simulink model "OFDM_Tx_HW"  (R2020a)
settings: Solver=FixedStepDiscrete  StartTime=0.0  StopTime=inf  RelTol=1e-3
InitFcn:
  | % Set parameters
  | fs = 20e6;
  | fclk = 240e6;
  | ssr = 2;
  | fdc = fclk*ssr*8;
  | 
  | % Load libraries
  | addpath('./lib');
  | 
  | % Create filters
  | run ./filter_design_20mhz;
  | 
  | % Load all required variables
  | load('variables/read_addr_data');
  | load('variables/read_addr_cp');
  | load('variables/read_addr_pream');
  | load('variables/read_addr_rx');
  | load('variables/pilot');
  | load('variables/sc_index');
  | load('variables/LTSfreq');
  | load('variables/STSfreq');
  | load('variables/LTSread');
  | load('variables/STSread');
  | 
  | run ./scripts/rfgen;
values from neighbouring files (symbols this model uses):
  decimation_unique = dsp.SampleRateConverter('InputSampleRate', fdc/64,     'OutputSampleRate', fs,     'Bandwidth', fs*0.9,     'OutputRateTolerance', 0,     'StopbandAttenuation', 100)    [filter_design_20mhz.m]
  interpolation_single = dsp.SampleRateConverter('InputSampleRate', fs,     'OutputSampleRate', fclk,     'Bandwidth', fs*0.9,     'OutputRateTolerance', 0,     'StopbandAttenuation', 100)    [filter_design_20mhz.m]
  interpolation_ssr = dsp.SampleRateConverter('InputSampleRate', fclk,     'OutputSampleRate', fclk*ssr,     'Bandwidth', fs*0.9,     'OutputRateTolerance', 0,     'StopbandAttenuation', 100)    [filter_design_20mhz.m]
undefined symbols (not defined in the file or in its folder): designMultirateFIR, LTSfreq, LTSread, pilot, read_addr_cp, read_addr_data, read_addr_pream, read_addr_rx, sc_index, STSfreq, STSread
libraries: hdlsllib x87, simulink x55, xbsIndex_r4 x48, dspmlti4 x23, xrbsSSR_Library x8, dspsigops x6, dspswit3 x4, dsphdlmathfun x3, dspsigattribs x2, dsphdlxfrm x2, dsphdlsigops x1, lib_rfsignalgenerator x1
(part 3 of 6)

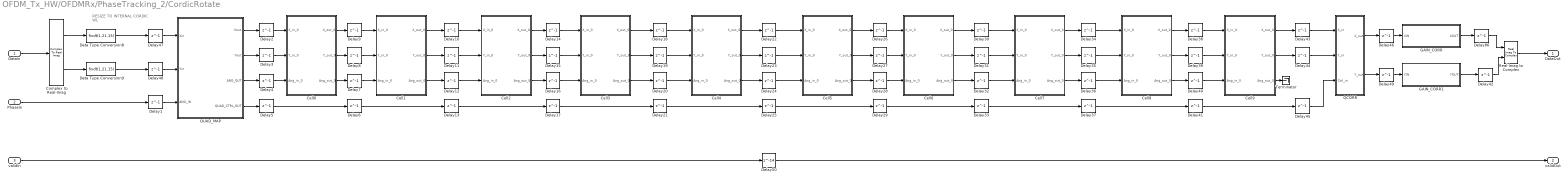
== system OFDM_Tx_HW/OFDMRx/PhaseTracking_2/CordicRotate ==
  note: RESIZE TO INTERNAL
      | CORDIC WL
  DataIn : Inport
  PhaseIn : Inport  Port=2
  validIn : Inport  Port=3
  Cell0 : Subsystem
  Cell1 : Subsystem
  Cell2 : Subsystem
  Cell3 : Subsystem
  Cell4 : Subsystem
  Cell5 : Subsystem
  Cell6 : Subsystem
  Cell7 : Subsystem
  Cell8 : Subsystem
  Cell9 : Subsystem
  Complex to Real-Imag : ComplexToRealImag
  Data Type Conversion8 : DataTypeConversion  OutDataTypeStr=fixdt(1,21,15)
  Data Type Conversion9 : DataTypeConversion  OutDataTypeStr=fixdt(1,21,15)
  Delay{1..49,86} (50 alike) : Delay  DelayLength=1
  Delay50 : Delay  DelayLength=14
  GAIN_CORR : Subsystem
  GAIN_CORR1 : Subsystem
  QCORR : Subsystem
  QUAD_MAP : Subsystem
  Real-Imag to Complex : RealImagToComplex
  Terminator : Terminator
  "DataOut  " : Outport  VectorParamsAs1DForOutWhenUnconnected=off
  validOut : Outport  Port=2  VectorParamsAs1DForOutWhenUnconnected=off
  wires:
  Delay50/1 -> validOut/1
  validIn/1 -> Delay50/1
  Real-Imag to Complex/1 -> "DataOut  "/1
  Delay42/1 -> Real-Imag to Complex/2
  Delay86/1 -> Real-Imag to Complex/1
  Complex to Real-Imag/1 -> Data Type Conversion8/1
  DataIn/1 -> Complex to Real-Imag/1
  Complex to Real-Imag/2 -> Data Type Conversion9/1
  GAIN_CORR/1(XOUT) -> Delay86/1
  Delay48/1 -> QUAD_MAP/2(Yin)
  Delay47/1 -> QUAD_MAP/1(Xin)
  QUAD_MAP/1(Xout) -> Delay2/1
  QUAD_MAP/2(Yout) -> Delay3/1
  QUAD_MAP/3(ANG_OUT) -> Delay4/1
  Delay2/1 -> Cell0/1(X_in_0)
  Delay3/1 -> Cell0/2(Y_in_0)
  QUAD_MAP/4(QUAD_CTRL_OUT) -> Delay5/1
  Cell0/1(X_out_0) -> Delay9/1
  Cell0/2(Y_out_0) -> Delay8/1
  Cell0/3(Ang_out_0) -> Delay7/1
  Delay5/1 -> Delay6/1
  Delay7/1 -> Cell1/3(Ang_in_0)
  Delay8/1 -> Cell1/2(Y_in_0)
  Delay9/1 -> Cell1/1(X_in_0)
  Cell1/1(X_out_0) -> Delay10/1
  Cell1/2(Y_out_0) -> Delay11/1
  Cell1/3(Ang_out_0) -> Delay12/1
  Delay6/1 -> Delay13/1
  Delay10/1 -> Cell2/1(X_in_0)
  Delay11/1 -> Cell2/2(Y_in_0)
  Delay12/1 -> Cell2/3(Ang_in_0)
  Delay16/1 -> Cell3/3(Ang_in_0)
  Delay15/1 -> Cell3/2(Y_in_0)
  Delay14/1 -> Cell3/1(X_in_0)
  Delay13/1 -> Delay17/1
  Cell2/3(Ang_out_0) -> Delay16/1
  Cell2/2(Y_out_0) -> Delay15/1
  Cell2/1(X_out_0) -> Delay14/1
  Cell3/1(X_out_0) -> Delay18/1
  Cell3/2(Y_out_0) -> Delay19/1
  Cell3/3(Ang_out_0) -> Delay20/1
  Delay17/1 -> Delay21/1
  Delay18/1 -> Cell4/1(X_in_0)
  Delay19/1 -> Cell4/2(Y_in_0)
  Delay20/1 -> Cell4/3(Ang_in_0)
  Delay24/1 -> Cell5/3(Ang_in_0)
  Delay23/1 -> Cell5/2(Y_in_0)
  Delay22/1 -> Cell5/1(X_in_0)
  Delay21/1 -> Delay25/1
  Cell4/3(Ang_out_0) -> Delay24/1
  Cell4/2(Y_out_0) -> Delay23/1
  Cell4/1(X_out_0) -> Delay22/1
  Cell5/1(X_out_0) -> Delay26/1
  Cell5/2(Y_out_0) -> Delay27/1
  Cell5/3(Ang_out_0) -> Delay28/1
  Delay25/1 -> Delay29/1
  Delay26/1 -> Cell6/1(X_in_0)
  Delay27/1 -> Cell6/2(Y_in_0)
  Delay28/1 -> Cell6/3(Ang_in_0)
  Delay32/1 -> Cell7/3(Ang_in_0)
  Delay31/1 -> Cell7/2(Y_in_0)
  Delay30/1 -> Cell7/1(X_in_0)
  Delay29/1 -> Delay33/1
  Cell6/3(Ang_out_0) -> Delay32/1
  Cell6/2(Y_out_0) -> Delay31/1
  Cell6/1(X_out_0) -> Delay30/1
  Cell7/1(X_out_0) -> Delay34/1
  Cell7/2(Y_out_0) -> Delay35/1
  Cell7/3(Ang_out_0) -> Delay36/1
  Delay33/1 -> Delay37/1
  Delay34/1 -> Cell8/1(X_in_0)
  Delay35/1 -> Cell8/2(Y_in_0)
  Delay36/1 -> Cell8/3(Ang_in_0)
  Delay40/1 -> Cell9/3(Ang_in_0)
  Delay39/1 -> Cell9/2(Y_in_0)
  Delay38/1 -> Cell9/1(X_in_0)
  Delay37/1 -> Delay41/1
  Cell8/3(Ang_out_0) -> Delay40/1
  Cell8/2(Y_out_0) -> Delay39/1
  Cell8/1(X_out_0) -> Delay38/1
  GAIN_CORR1/1(YOUT) -> Delay42/1
  Cell9/3(Ang_out_0) -> Terminator/1
  Delay41/1 -> Delay45/1
  Cell9/1(X_out_0) -> Delay43/1
  Cell9/2(Y_out_0) -> Delay44/1
  Delay43/1 -> QCORR/1(X_in)
  Delay44/1 -> QCORR/2(Y_in)
  Delay46/1 -> GAIN_CORR/1(XIN)
  Delay49/1 -> GAIN_CORR1/1(YIN)
  QCORR/2(Y_out) -> Delay49/1
  Delay1/1 -> QUAD_MAP/3(ANG_IN)
  Delay4/1 -> Cell0/3(Ang_in_0)
  Delay45/1 -> QCORR/3(Ctrl_in)
  Data Type Conversion8/1 -> Delay47/1
  Data Type Conversion9/1 -> Delay48/1
  PhaseIn/1 -> Delay1/1
  QCORR/1(X_out) -> Delay46/1

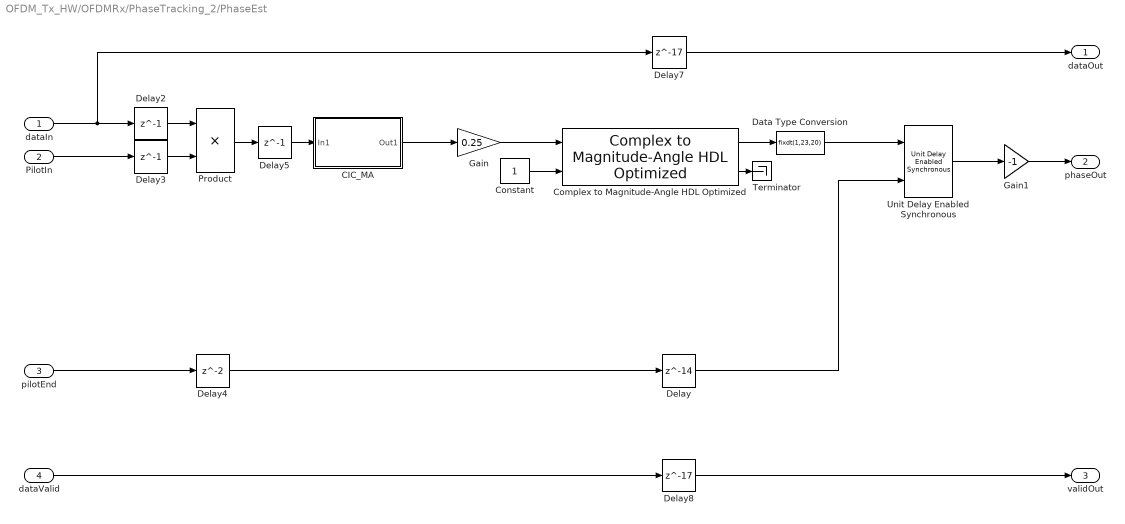
== system OFDM_Tx_HW/OFDMRx/PhaseTracking_2/PhaseEst ==
  dataIn : Inport
  PilotIn : Inport  Port=2
  pilotEnd : Inport  Port=3
  dataValid : Inport  Port=4
  CIC_MA : Subsystem
  Complex to Magnitude-Angle HDL Optimized : dsphdlmathfun/Complex to Magnitude-Angle HDL Optimized  NumIterationsSource=Property  NumIterations=10  OutputFormat=Angle  AngleFormat=Radians  ScaleOutput=off  SimulateUsing=Code generation
      settings: SourceProductBaseCode=DS
  Constant : Constant  OutDataTypeStr=boolean  SampleTime=1/fs
  Data Type Conversion : DataTypeConversion  OutDataTypeStr=fixdt(1,23,20)
  Delay : Delay  DelayLength=14
  Delay2 : Delay  DelayLength=1
  Delay3 : Delay  DelayLength=1
  Delay4 : Delay
  Delay5 : Delay  DelayLength=1
  Delay7 : Delay  DelayLength=17
  Delay8 : Delay  DelayLength=17
  Gain : Gain  Gain=0.25  OutDataTypeStr=fixdt(1,18,15)
  Gain1 : Gain  Gain=-1  OutDataTypeStr=fixdt(1,23,20)
  Product : Product  OutDataTypeStr=fixdt(1,18,15)
  Terminator : Terminator
  Unit Delay Enabled Synchronous : hdlsllib/Discrete/Unit Delay Enabled Synchronous  InitialCondition=0.0  SampleTime=-1
      settings: SourceProductBaseCode=SL
  dataOut : Outport  VectorParamsAs1DForOutWhenUnconnected=off
  phaseOut : Outport  Port=2  VectorParamsAs1DForOutWhenUnconnected=off
  validOut : Outport  Port=3  VectorParamsAs1DForOutWhenUnconnected=off
  wires:
  Data Type Conversion/1 -> Unit Delay Enabled Synchronous/1
  Gain1/1 -> phaseOut/1
  Delay4/1 -> Delay/1
  Complex to Magnitude-Angle HDL Optimized/2 -> Terminator/1
  Complex to Magnitude-Angle HDL Optimized/1 -> Data Type Conversion/1
  Gain/1 -> Complex to Magnitude-Angle HDL Optimized/1
  Constant/1 -> Complex to Magnitude-Angle HDL Optimized/2
  Delay8/1 -> validOut/1
  Unit Delay Enabled Synchronous/1 -> Gain1/1
  Delay7/1 -> dataOut/1
  dataValid/1 -> Delay8/1
  pilotEnd/1 -> Delay4/1
  Delay5/1 -> CIC_MA/1(In1)
  Delay3/1 -> Product/2
  Delay2/1 -> Product/1
  Product/1 -> Delay5/1
  dataIn/1 -> Delay2/1, Delay7/1
  PilotIn/1 -> Delay3/1
  Delay/1 -> Unit Delay Enabled Synchronous/2
  CIC_MA/1(Out1) -> Gain/1

== system OFDM_Tx_HW/OFDMRx/PhaseTracking_2/PilotCtrlGen ==
  dataIn : Inport
  ValidIn : Inport  Port=2
  CtrlSigGen : Subsystem
  Delay1 : Delay  DelayLength=1
  Delay10 : Delay  DelayLength=1
  SampleCounter : Subsystem
  SymbolCounter : Subsystem
  pilotGen : Subsystem
  dataOut : Outport  VectorParamsAs1DForOutWhenUnconnected=off
  pilotOut : Outport  Port=2  VectorParamsAs1DForOutWhenUnconnected=off
  PilotEnd : Outport  Port=3  VectorParamsAs1DForOutWhenUnconnected=off
  dataValid : Outport  Port=4  VectorParamsAs1DForOutWhenUnconnected=off
  wires:
  Delay1/1 -> pilotGen/3(valid), CtrlSigGen/1(valid)
  SampleCounter/1(Sample_Cnt) -> pilotGen/2(sampleCount), CtrlSigGen/2(sampleCount)
  CtrlSigGen/2(pilotEnd) -> PilotEnd/1
  CtrlSigGen/1(dataValid) -> dataValid/1
  SymbolCounter/1(Symbl_cnt) -> pilotGen/1(symbCount)
  ValidIn/1 -> SymbolCounter/1(ValidIn), SampleCounter/1(Valid_In), Delay1/1
  pilotGen/1(pilOut) -> pilotOut/1
  Delay10/1 -> dataOut/1
  dataIn/1 -> Delay10/1

== system OFDM_Tx_HW/OFDMRx/Synchronisation/CoarseFreqCorr ==
  note: Reccord the phase of the averaged autocorrelation at the coarse
      | timing point.
  note: Correct frequency offset
  note: Generate complex sinusoid with a frequency equal
      | to the estimated frequency offset.
  dataIn : Inport
  frameDet : Inport  Port=2
  phaseIn : Inport  Port=3
  Constant : Constant  VectorParams1D=off  OutDataTypeStr=boolean  SampleTime=1/fs
  Delay{,2,5,7} (4 alike) : Delay  DelayLength=1
  Delay1 : Delay  DelayLength=9
  Delay3 : Delay  DelayLength=6
  Gain : Gain  Gain=2048  OutDataTypeStr=uint16
  Math Function : Math  Operator=conj  SignedPower=on  RndMeth=Zero  SaturateOnIntegerOverflow=on
  NCO HDL Optimized : dsphdlsigops/NCO HDL Optimized  PhaseIncrementSource=Input port  PhaseIncrement=100  PhaseOffsetSource=Property  PhaseOffset=0  DitherSource=Property  NumDitherBits=4  SamplesPerFrame=1  LUTCompress=on  ResetAction=off  Waveform=Complex exponential  PhasePort=off  SimulateUsing=Code generation  AccumulatorWL=16  PhaseQuantization=on  NumQuantizerAccumulatorBits=12  OutputDataType=Binary point scaling  OutputWL=16  OutputFL=14
      settings: SourceProductBaseCode=DS
  Product : Product  OutDataTypeStr=fixdt(1,16,14)
  RsingEdge : Subsystem
  Terminator : Terminator
  Unit Delay Enabled Synchronous : hdlsllib/Discrete/Unit Delay Enabled Synchronous  InitialCondition=0.0  SampleTime=-1
      settings: SourceProductBaseCode=SL
  dataOut : Outport  VectorParamsAs1DForOutWhenUnconnected=off
  frameDetOut : Outport  Port=2  VectorParamsAs1DForOutWhenUnconnected=off
  wires:
  Delay7/1 -> dataOut/1
  Delay1/1 -> frameDetOut/1
  Math Function/1 -> Delay5/1
  Delay3/1 -> Delay/1
  Product/1 -> Delay7/1
  Delay5/1 -> Product/2
  Delay/1 -> Product/1
  dataIn/1 -> Delay2/1
  phaseIn/1 -> Unit Delay Enabled Synchronous/1
  RsingEdge/1(Out1) -> Unit Delay Enabled Synchronous/2
  frameDet/1 -> Delay1/1, RsingEdge/1(In1)
  Delay2/1 -> Delay3/1
  Unit Delay Enabled Synchronous/1 -> Gain/1
  Gain/1 -> NCO HDL Optimized/1
  NCO HDL Optimized/1 -> Math Function/1
  NCO HDL Optimized/2 -> Terminator/1
  Constant/1 -> NCO HDL Optimized/2

== system OFDM_Tx_HW/OFDMRx/Synchronisation/ControlSigGen ==
  validIn : Inport
  OR : Logic  Operator=OR  IconShape=distinctive  AllPortsSameDT=off  OutDataTypeStr=boolean
  PreambleValidGen : Subsystem
  dataValidGen : Subsystem
  FFTValid : Outport  VectorParamsAs1DForOutWhenUnconnected=off
  dataValid : Outport  Port=2  VectorParamsAs1DForOutWhenUnconnected=off
  preambleValid : Outport  Port=3  VectorParamsAs1DForOutWhenUnconnected=off
  wires:
  OR/1 -> FFTValid/1
  dataValidGen/1(y) -> dataValid/1, OR/2
  PreambleValidGen/1(y) -> dataValidGen/1(enb), OR/1, preambleValid/1
  validIn/1 -> PreambleValidGen/1(ValidIn), dataValidGen/2(enb1)

== system OFDM_Tx_HW/OFDMRx/Synchronisation/Delay ==
  note: Delay coarse timing point from middle of L-STF
      | to beginning of 1st repetition of L-LTF
  data : Inport
  strobe : Inport  Port=2
  Delay3 : Delay  DelayLength=108  InputProcessing=Columns as channels (frame based)
  dataOut : Outport
  strobeOut : Outport  Port=2
  wires:
  data/1 -> dataOut/1
  Delay3/1 -> strobeOut/1
  strobe/1 -> Delay3/1

== system OFDM_Tx_HW/OFDMRx/Synchronisation/FrameDetect ==
  note: The frame is detected when the timing metric exceeds the threshold for 30 successive samples. This
      | corresponds to the coarse timing point, which should occur in the middle of the L-STF.
  leftIn : Inport
  rightIn : Inport  Port=2
  phaseIn : Inport  Port=3
  Compare To Constant : simulink/Logic and Bit Operations/Compare To Constant  relop===  const=29  OutDataTypeStr=boolean
  Delay{,2..4} (4 alike) : Delay  DelayLength=1
  HDL Counter : hdlsllib/Sources/HDL Counter  CountType=Count limited  CountInit=0  CountStep=1  CountMax=29  CountFromType=Initial value  CountFrom=0  CountResetPort=on  CountLoadPort=off  CountEnbPort=on  CountDirPort=off  CountDataType=Unsigned  CountWordLen=5  CountFracLen=0  CountSampTime=1
  Logical Operator : Logic  Operator=OR  IconShape=distinctive  AllPortsSameDT=off  OutDataTypeStr=boolean
  Logical Operator1 : Logic  Operator=NOT  IconShape=distinctive  AllPortsSameDT=off  OutDataTypeStr=boolean
  Relational Operator : RelationalOperator  Operator=>  OutDataTypeStr=boolean  RndMeth=Simplest
  RsingEdge : Subsystem
  frameDet : Outport  VectorParamsAs1DForOutWhenUnconnected=off
  phaseOut : Outport  Port=2  VectorParamsAs1DForOutWhenUnconnected=off
  wires:
  Delay3/1 -> Relational Operator/2
  Relational Operator/1 -> HDL Counter/2, Logical Operator1/1
  Logical Operator1/1 -> Logical Operator/2
  rightIn/1 -> Delay3/1
  HDL Counter/1 -> Compare To Constant/1
  Compare To Constant/1 -> RsingEdge/1(In1), Logical Operator/1
  Logical Operator/1 -> HDL Counter/1
  phaseIn/1 -> Delay4/1
  leftIn/1 -> Delay2/1
  Delay/1 -> phaseOut/1
  RsingEdge/1(Out1) -> frameDet/1
  Delay2/1 -> Relational Operator/1
  Delay4/1 -> Delay/1

== system OFDM_Tx_HW/OFDMRx/Synchronisation/SchmidlCoxMetric  ==
  note: The Schmidl & Cox timing metric is used for frame detection. The timing metric, M(d), is compared to a threshold
      | to determine if a frame is present. In order to avoid division, we re-arrange the timing metric as |P(d)|^2 > (R(d))^2 x thresh.
      | The phase of the averaged autocorrelation is also determined for Carrier Frequency Offset (CFO) estimation purposes.
  note: |P(d)|^2
  note: (R(d))^2 x thresh
  dataIn : Inport
  threshold : Inport  Port=2
  Abs2 : Subsystem
  AutoCorr : Subsystem
  CIC_ma : Subsystem
  CIC_ma1 : Subsystem
  Data Type Conversion : DataTypeConversion  OutDataTypeStr=fixdt(0,32,31)  ConvertRealWorld=Stored Integer (SI)
  Delay : Delay  DelayLength=14
  Delay2 : Delay
  MagPhase : Subsystem
  Sq : Subsystem
  Sq1 : Subsystem
  ThreshMult : Subsystem
  left : Outport  VectorParamsAs1DForOutWhenUnconnected=off
  right : Outport  Port=2  VectorParamsAs1DForOutWhenUnconnected=off
  phase : Outport  Port=3  VectorParamsAs1DForOutWhenUnconnected=off
  wires:
  threshold/1 -> Data Type Conversion/1
  Data Type Conversion/1 -> ThreshMult/2(threshold)
  Sq/1(Out1) -> left/1
  ThreshMult/1(Out1) -> right/1
  Sq1/1(Out1) -> ThreshMult/1(In1)
  Delay/1 -> Sq1/1(In1)
  CIC_ma1/1(Out1) -> Delay/1
  dataIn/1 -> AutoCorr/1(AcorrIn), Abs2/1(Abs2In)
  Abs2/1(Abs2Out) -> CIC_ma1/1(In1)
  MagPhase/2(Mag) -> Sq/1(In1)
  AutoCorr/1(AcorrOut) -> CIC_ma/1(In1)
  CIC_ma/1(Out1) -> MagPhase/1(dataIn)
  Delay2/1 -> phase/1
  MagPhase/1(Phase) -> Delay2/1

== system OFDM_Tx_HW/OFDMTx/CPAdd/DataExtend ==
  dataIn : Inport
  dataValid : Inport  Port=2
  Delay1 : Delay  DelayLength=80  InitialCondition=0  UseCircularBuffer=on
  Delay2 : Delay  DelayLength=80
  Delay3 : Delay  DelayLength=1  InitialCondition=0  UseCircularBuffer=on
  Delay4 : Delay  DelayLength=80
  Dual Port RAM2 : hdlsllib/HDL RAMs/Dual Port RAM  ram_size=8
      settings: SourceProductBaseCode=SL
  HDL Counter : hdlsllib/Sources/HDL Counter  CountType=Count limited  CountInit=0  CountStep=1  CountMax=159  CountFromType=Initial value  CountFrom=0  CountResetPort=off  CountLoadPort=off  CountEnbPort=on  CountDirPort=off  CountDataType=Unsigned  CountWordLen=8  CountFracLen=0  CountSampTime=1
  HDL Counter1 : hdlsllib/Sources/HDL Counter  CountType=Count limited  CountInit=0  CountStep=1  CountMax=159  CountFromType=Initial value  CountFrom=0  CountResetPort=off  CountLoadPort=off  CountEnbPort=on  CountDirPort=off  CountDataType=Unsigned  CountWordLen=8  CountFracLen=0  CountSampTime=1
  READ_ADDRESS : Lookup_n-D  NumberOfTableDimensions=1  LookupTableObject=''  BreakpointsForDimension1=[0:159]  BreakpointsForDimension1FirstPoint=10  BreakpointsForDimension2FirstPoint=10  BreakpointsForDimension1Spacing=12  BreakpointsForDimension2Spacing=12  IndexSearchMethod=Evenly spaced points  Table=read_addr_cp  TableDataTypeStr=fixdt(0,8,0)  InterpMethod=Flat  DiagnosticForOutOfRangeInput=Error  InternalRulePriority=Speed  OutDataTypeStr=fixdt(0,8,0)  RndMeth=Simplest  InputSameDT=on
  READ_CTRL2 : Subsystem
  Terminator3 : Terminator
  dataOut : Outport  VectorParamsAs1DForOutWhenUnconnected=off
  dataValidOut : Outport  Port=2  VectorParamsAs1DForOutWhenUnconnected=off
  wires:
  Delay4/1 -> dataOut/1
  Delay2/1 -> dataValidOut/1
  Dual Port RAM2/1 -> Terminator3/1
  READ_ADDRESS/1 -> READ_CTRL2/1(In1)
  HDL Counter/1 -> READ_ADDRESS/1
  dataIn/1 -> Dual Port RAM2/1
  HDL Counter1/1 -> Dual Port RAM2/2
  Delay1/1 -> HDL Counter/1, Delay3/1, READ_CTRL2/2(In2)
  Dual Port RAM2/2 -> Delay4/1
  dataValid/1 -> HDL Counter1/1, Dual Port RAM2/3, Delay1/1
  Delay3/1 -> Delay2/1
  READ_CTRL2/1(Out1) -> Dual Port RAM2/4

== system OFDM_Tx_HW/OFDMTx/CPAdd/LTFExtend ==
  data : Inport
  preambVal : Inport  Port=2
  Delay : Delay  DelayLength=160  InitialCondition=0  UseCircularBuffer=on
  Delay12 : Delay  DelayLength=1  InitialCondition=0  UseCircularBuffer=on
  Dual Port RAM : hdlsllib/HDL RAMs/Dual Port RAM  ram_size=8
      settings: SourceProductBaseCode=SL
  HDL Counter2 : hdlsllib/Sources/HDL Counter  CountType=Count limited  CountInit=0  CountStep=1  CountMax=159  CountFromType=Initial value  CountFrom=0  CountResetPort=off  CountLoadPort=off  CountEnbPort=on  CountDirPort=off  CountDataType=Unsigned  CountWordLen=8  CountFracLen=0  CountSampTime=1
  HDL Counter3 : hdlsllib/Sources/HDL Counter  CountType=Count limited  CountInit=0  CountStep=1  CountMax=159  CountFromType=Initial value  CountFrom=0  CountResetPort=off  CountLoadPort=off  CountEnbPort=on  CountDirPort=off  CountDataType=Unsigned  CountWordLen=8  CountFracLen=0  CountSampTime=1
  LTFValidGen : Subsystem
  READ_CTRL : Subsystem
  Terminator1 : Terminator
  readaddr : Lookup_n-D  NumberOfTableDimensions=1  LookupTableObject=''  BreakpointsForDimension1=0:159  BreakpointsForDimension1FirstPoint=10  BreakpointsForDimension2FirstPoint=10  BreakpointsForDimension1Spacing=12  BreakpointsForDimension2Spacing=12  IndexSearchMethod=Evenly spaced points  Table=LTSread  TableDataTypeStr=fixdt(0,8,0)  InterpMethod=Flat  DiagnosticForOutOfRangeInput=Error  InternalRulePriority=Speed  OutDataTypeStr=fixdt(0,8,0)  RndMeth=Simplest  InputSameDT=on
  LTFExtendOut : Outport  VectorParamsAs1DForOutWhenUnconnected=off
  LTFValidOut : Outport  Port=2  VectorParamsAs1DForOutWhenUnconnected=off
  wires:
  readaddr/1 -> READ_CTRL/1(In1)
  READ_CTRL/1(Out1) -> Dual Port RAM/4
  HDL Counter3/1 -> Dual Port RAM/2
  Delay/1 -> READ_CTRL/2(In2), Delay12/1, HDL Counter2/1
  Dual Port RAM/1 -> Terminator1/1
  Delay12/1 -> LTFValidOut/1
  HDL Counter2/1 -> readaddr/1
  data/1 -> Dual Port RAM/1
  Dual Port RAM/2 -> LTFExtendOut/1
  preambVal/1 -> LTFValidGen/1(In1)
  LTFValidGen/1(Out1) -> Dual Port RAM/3, Delay/1, HDL Counter3/1

== system OFDM_Tx_HW/OFDMTx/CPAdd/STFExtend ==
  data : Inport
  preambVal : Inport  Port=2
  Delay : Delay  DelayLength=160  InitialCondition=0  UseCircularBuffer=on
  Delay12 : Delay  DelayLength=1  InitialCondition=0  UseCircularBuffer=on
  Dual Port RAM : hdlsllib/HDL RAMs/Dual Port RAM  ram_size=8
      settings: SourceProductBaseCode=SL
  HDL Counter2 : hdlsllib/Sources/HDL Counter  CountType=Count limited  CountInit=0  CountStep=1  CountMax=159  CountFromType=Initial value  CountFrom=0  CountResetPort=off  CountLoadPort=off  CountEnbPort=on  CountDirPort=off  CountDataType=Unsigned  CountWordLen=8  CountFracLen=0  CountSampTime=1
  HDL Counter3 : hdlsllib/Sources/HDL Counter  CountType=Count limited  CountInit=0  CountStep=1  CountMax=159  CountFromType=Initial value  CountFrom=0  CountResetPort=off  CountLoadPort=off  CountEnbPort=on  CountDirPort=off  CountDataType=Unsigned  CountWordLen=8  CountFracLen=0  CountSampTime=1
  READ_CTRL : Subsystem
  STFValidGen : Subsystem
  Terminator1 : Terminator
  readaddr : Lookup_n-D  NumberOfTableDimensions=1  LookupTableObject=''  BreakpointsForDimension1=0:159  BreakpointsForDimension1FirstPoint=10  BreakpointsForDimension2FirstPoint=10  BreakpointsForDimension1Spacing=12  BreakpointsForDimension2Spacing=12  IndexSearchMethod=Evenly spaced points  Table=STSread  TableDataTypeStr=fixdt(0,8,0)  InterpMethod=Flat  DiagnosticForOutOfRangeInput=Error  InternalRulePriority=Speed  OutDataTypeStr=fixdt(0,8,0)  RndMeth=Simplest  InputSameDT=on
  STFExtendOut : Outport  VectorParamsAs1DForOutWhenUnconnected=off
  STFValidOut : Outport  Port=2  VectorParamsAs1DForOutWhenUnconnected=off
  wires:
  Dual Port RAM/2 -> STFExtendOut/1
  data/1 -> Dual Port RAM/1
  HDL Counter2/1 -> readaddr/1
  Delay12/1 -> STFValidOut/1
  Dual Port RAM/1 -> Terminator1/1
  Delay/1 -> HDL Counter2/1, Delay12/1, READ_CTRL/2(In2)
  HDL Counter3/1 -> Dual Port RAM/2
  READ_CTRL/1(Out1) -> Dual Port RAM/4
  preambVal/1 -> STFValidGen/1(In1)
  readaddr/1 -> READ_CTRL/1(In1)
  STFValidGen/1(Out1) -> HDL Counter3/1, Dual Port RAM/3, Delay/1

== system OFDM_Tx_HW/OFDMTx/ControlSignalGenerator/PreamValidGen ==
  enable : Inport
  Compare To Constant : simulink/Logic and Bit Operations/Compare To Constant  relop===  const=320  OutDataTypeStr=boolean
  HDL Counter : hdlsllib/Sources/HDL Counter  CountType=Count limited  CountInit=0  CountStep=1  CountMax=320  CountFromType=Initial value  CountFrom=0  CountResetPort=on  CountLoadPort=off  CountEnbPort=on  CountDirPort=off  CountDataType=Unsigned  CountWordLen=9  CountFracLen=0  CountSampTime=1
  NOT : Logic  Operator=NOT  IconShape=distinctive  AllPortsSameDT=off  OutDataTypeStr=boolean
  RisingEdge : Subsystem
  Unit Delay Enabled Resettable Synchronous : hdlsllib/Discrete/Unit Delay Enabled Resettable Synchronous  InitialCondition=0.0  SampleTime=-1
      settings: SourceProductBaseCode=SL
  y : Outport  VectorParamsAs1DForOutWhenUnconnected=off
  wires:
  HDL Counter/1 -> Compare To Constant/1
  RisingEdge/1(Out1) -> Unit Delay Enabled Resettable Synchronous/2
  Compare To Constant/1 -> Unit Delay Enabled Resettable Synchronous/3
  enable/1 -> RisingEdge/1(In1), Unit Delay Enabled Resettable Synchronous/1, NOT/1, HDL Counter/2
  Unit Delay Enabled Resettable Synchronous/1 -> y/1
  NOT/1 -> HDL Counter/1

== system OFDM_Tx_HW/OFDMTx/ControlSignalGenerator/dataReadyGen ==
  enb : Inport
  Compare To Constant : simulink/Logic and Bit Operations/Compare To Constant  relop=>  const=31  OutDataTypeStr=boolean
  HDL Counter : hdlsllib/Sources/HDL Counter  CountType=Count limited  CountInit=0  CountStep=1  CountMax=79  CountFromType=Initial value  CountFrom=0  CountResetPort=on  CountLoadPort=off  CountEnbPort=on  CountDirPort=off  CountDataType=Unsigned  CountWordLen=7  CountFracLen=0  CountSampTime=1
  NOT : Logic  Operator=NOT  IconShape=distinctive  AllPortsSameDT=off  OutDataTypeStr=boolean
  y : Outport
  wires:
  HDL Counter/1 -> Compare To Constant/1
  enb/1 -> NOT/1, HDL Counter/2
  NOT/1 -> HDL Counter/1
  Compare To Constant/1 -> y/1

== system OFDM_Tx_HW/OFDMTx/ControlSignalGenerator/dataValidGen ==
  y : Inport
  enable : Inport  Port=2
  AND : Logic  IconShape=distinctive  AllPortsSameDT=off  OutDataTypeStr=boolean
  Delay : Delay  DelayLength=1
  NOT : Logic  Operator=NOT  IconShape=distinctive  AllPortsSameDT=off  OutDataTypeStr=boolean
  valOut : Outport
  wires:
  NOT/1 -> AND/1
  Delay/1 -> AND/2
  AND/1 -> valOut/1
  y/1 -> NOT/1
  enable/1 -> Delay/1

== system OFDM_Tx_HW/OFDMTx/ControlSignalGenerator/pilotValidGen ==
  enb : Inport
  AND : Logic  IconShape=distinctive  AllPortsSameDT=off  OutDataTypeStr=boolean
  Compare To Constant : simulink/Logic and Bit Operations/Compare To Constant  relop=<  const=32  OutDataTypeStr=boolean
  Compare To Constant1 : simulink/Logic and Bit Operations/Compare To Constant  relop=>  const=27  OutDataTypeStr=boolean
  HDL Counter : hdlsllib/Sources/HDL Counter  CountType=Count limited  CountInit=0  CountStep=1  CountMax=79  CountFromType=Initial value  CountFrom=0  CountResetPort=on  CountLoadPort=off  CountEnbPort=on  CountDirPort=off  CountDataType=Unsigned  CountWordLen=7  CountFracLen=0  CountSampTime=1
  NOT : Logic  Operator=NOT  IconShape=distinctive  AllPortsSameDT=off  OutDataTypeStr=boolean
  y : Outport
  wires:
  NOT/1 -> HDL Counter/1
  enb/1 -> HDL Counter/2, NOT/1
  HDL Counter/1 -> Compare To Constant1/1, Compare To Constant/1
  Compare To Constant/1 -> AND/1
  Compare To Constant1/1 -> AND/2
  AND/1 -> y/1

== system OFDM_Tx_HW/OFDMTx/DataGenerator/LTSfreq ==
  preambVal : Inport
  AND : Logic  IconShape=distinctive  AllPortsSameDT=off  OutDataTypeStr=boolean
  AND1 : Logic  IconShape=distinctive  AllPortsSameDT=off  OutDataTypeStr=boolean
  Compare To Constant : simulink/Logic and Bit Operations/Compare To Constant  relop=>=  const=256  OutDataTypeStr=boolean
  Compare To Constant1 : simulink/Logic and Bit Operations/Compare To Constant  relop=<=  const=319  OutDataTypeStr=boolean
  HDL Counter1 : hdlsllib/Sources/HDL Counter  CountType=Count limited  CountInit=0  CountStep=1  CountMax=319  CountFromType=Initial value  CountFrom=0  CountResetPort=on  CountLoadPort=off  CountEnbPort=on  CountDirPort=off  CountDataType=Unsigned  CountWordLen=9  CountFracLen=0  CountSampTime=1
  HDL Counter4 : hdlsllib/Sources/HDL Counter  CountType=Count limited  CountInit=0  CountStep=1  CountMax=63  CountFromType=Initial value  CountFrom=0  CountResetPort=off  CountLoadPort=off  CountEnbPort=on  CountDirPort=off  CountDataType=Unsigned  CountWordLen=6  CountFracLen=0  CountSampTime=1
  LTSFreq : Lookup_n-D  NumberOfTableDimensions=1  LookupTableObject=''  BreakpointsForDimension1=0:63  BreakpointsForDimension1FirstPoint=10  BreakpointsForDimension2FirstPoint=10  BreakpointsForDimension1Spacing=12  BreakpointsForDimension2Spacing=12  IndexSearchMethod=Evenly spaced points  Table=LTSfreq  TableDataTypeStr=fixdt(1,16,14)  InterpMethod=Flat  DiagnosticForOutOfRangeInput=Error  InternalRulePriority=Speed  OutDataTypeStr=fixdt(1,16,14)  RndMeth=Simplest  InputSameDT=on
  NOT : Logic  Operator=NOT  IconShape=distinctive  AllPortsSameDT=off  OutDataTypeStr=boolean
  ltsFreq : Outport  VectorParamsAs1DForOutWhenUnconnected=off
  ltsVal : Outport  Port=2  VectorParamsAs1DForOutWhenUnconnected=off
  wires:
  HDL Counter4/1 -> LTSFreq/1
  Compare To Constant/1 -> AND/1
  HDL Counter1/1 -> Compare To Constant1/1, Compare To Constant/1
  Compare To Constant1/1 -> AND/2
  NOT/1 -> HDL Counter1/1
  AND/1 -> AND1/1
  preambVal/1 -> NOT/1, AND1/2, HDL Counter1/2
  AND1/1 -> ltsVal/1, HDL Counter4/1
  LTSFreq/1 -> ltsFreq/1

== system OFDM_Tx_HW/OFDMTx/DataGenerator/PilotGen ==
  dataValidIn : Inport
  pilotValidIn : Inport  Port=2
  Compare To Constant : simulink/Logic and Bit Operations/Compare To Constant  relop=>  const=0  OutDataTypeStr=boolean
  Compare To Constant1 : simulink/Logic and Bit Operations/Compare To Constant  relop===  const=79  OutDataTypeStr=boolean
  Constant : Constant  Value=0  OutDataTypeStr=fixdt(1,2,0)  SampleTime=1/fs
  Data Type Conversion1 : DataTypeConversion  OutDataTypeStr=fixdt(1,16,14)
  HDL Counter : hdlsllib/Sources/HDL Counter  CountType=Count limited  CountInit=0  CountStep=1  CountMax=3  CountFromType=Initial value  CountFrom=0  CountResetPort=off  CountLoadPort=off  CountEnbPort=on  CountDirPort=off  CountDataType=Unsigned  CountWordLen=2  CountFracLen=0  CountSampTime=1
  HDL Counter1 : hdlsllib/Sources/HDL Counter  CountType=Count limited  CountInit=0  CountStep=1  CountMax=79  CountFromType=Initial value  CountFrom=0  CountResetPort=on  CountLoadPort=off  CountEnbPort=on  CountDirPort=off  CountDataType=Unsigned  CountWordLen=8  CountFracLen=0  CountSampTime=1
  HDL Counter2 : hdlsllib/Sources/HDL Counter  CountType=Count limited  CountInit=0  CountStep=1  CountMax=126  CountFromType=Initial value  CountFrom=0  CountResetPort=on  CountLoadPort=off  CountEnbPort=on  CountDirPort=off  CountDataType=Unsigned  CountWordLen=7  CountFracLen=0  CountSampTime=1
  NOT : Logic  Operator=NOT  IconShape=distinctive  AllPortsSameDT=off  OutDataTypeStr=boolean
  PilotValue_LUT : Lookup_n-D  NumberOfTableDimensions=1  LookupTableObject=''  BreakpointsForDimension1=[0:3]  BreakpointsForDimension1FirstPoint=10  BreakpointsForDimension2FirstPoint=10  BreakpointsForDimension1Spacing=12  BreakpointsForDimension2Spacing=12  IndexSearchMethod=Evenly spaced points  Table=[1 1 1 -1]  TableDataTypeStr=fixdt(1,2,0)  InterpMethod=Flat  DiagnosticForOutOfRangeInput=Error  InternalRulePriority=Speed  OutDataTypeStr=fixdt(1,2,0)  RndMeth=Simplest  InputSameDT=on
  Polarity_LUT : Lookup_n-D  NumberOfTableDimensions=1  LookupTableObject=''  BreakpointsForDimension1=[0:126]  BreakpointsForDimension1FirstPoint=10  BreakpointsForDimension2FirstPoint=10  BreakpointsForDimension1Spacing=12  BreakpointsForDimension2Spacing=12  IndexSearchMethod=Evenly spaced points  Table=pilot  TableDataTypeStr=fixdt(1,2,0)  InterpMethod=Flat  DiagnosticForOutOfRangeInput=Error  InternalRulePriority=Speed  OutDataTypeStr=fixdt(1,2,0)  RndMeth=Simplest  InputSameDT=on
  Switch : Switch  Criteria=u2 ~= 0
  Switch1 : Switch  Criteria=u2 ~= 0
  ToComplex1 : Subsystem
  Unary Minus : UnaryMinus
  pilotOut : Outport  VectorParamsAs1DForOutWhenUnconnected=off
  wires:
  HDL Counter/1 -> PilotValue_LUT/1
  Data Type Conversion1/1 -> ToComplex1/1(In1)
  dataValidIn/1 -> HDL Counter1/2, NOT/1
  HDL Counter1/1 -> Compare To Constant1/1
  NOT/1 -> HDL Counter2/1, HDL Counter1/1
  Compare To Constant1/1 -> HDL Counter2/2
  HDL Counter2/1 -> Polarity_LUT/1
  ToComplex1/1(PilotOut) -> pilotOut/1
  pilotValidIn/1 -> HDL Counter/1, Switch1/2
  Polarity_LUT/1 -> Compare To Constant/1
  Compare To Constant/1 -> Switch/2
  Unary Minus/1 -> Switch/3
  Switch/1 -> Data Type Conversion1/1
  PilotValue_LUT/1 -> Switch1/1
  Switch1/1 -> Unary Minus/1, Switch/1
  Constant/1 -> Switch1/3

== system OFDM_Tx_HW/OFDMTx/DataGenerator/STSFreq ==
  preamVal : Inport
  AND : Logic  IconShape=distinctive  AllPortsSameDT=off  OutDataTypeStr=boolean
  AND1 : Logic  IconShape=distinctive  AllPortsSameDT=off  OutDataTypeStr=boolean
  Compare To Constant : simulink/Logic and Bit Operations/Compare To Constant  relop=>=  const=96  OutDataTypeStr=boolean
  Compare To Constant1 : simulink/Logic and Bit Operations/Compare To Constant  relop=<=  const=159  OutDataTypeStr=boolean
  HDL Counter : hdlsllib/Sources/HDL Counter  CountType=Count limited  CountInit=0  CountStep=1  CountMax=63  CountFromType=Initial value  CountFrom=0  CountResetPort=off  CountLoadPort=off  CountEnbPort=on  CountDirPort=off  CountDataType=Unsigned  CountWordLen=6  CountFracLen=0  CountSampTime=1
  HDL Counter1 : hdlsllib/Sources/HDL Counter  CountType=Count limited  CountInit=0  CountStep=1  CountMax=319  CountFromType=Initial value  CountFrom=0  CountResetPort=on  CountLoadPort=off  CountEnbPort=on  CountDirPort=off  CountDataType=Unsigned  CountWordLen=9  CountFracLen=0  CountSampTime=1
  NOT : Logic  Operator=NOT  IconShape=distinctive  AllPortsSameDT=off  OutDataTypeStr=boolean
  STSFreq : Lookup_n-D  NumberOfTableDimensions=1  LookupTableObject=''  BreakpointsForDimension1=[0:63]  BreakpointsForDimension1FirstPoint=10  BreakpointsForDimension2FirstPoint=10  BreakpointsForDimension1Spacing=12  BreakpointsForDimension2Spacing=12  IndexSearchMethod=Evenly spaced points  Table=STSfreq  TableDataTypeStr=fixdt(1,16,14)  InterpMethod=Flat  DiagnosticForOutOfRangeInput=Error  InternalRulePriority=Speed  OutDataTypeStr=fixdt(1,16,14)  RndMeth=Simplest  InputSameDT=on
  stsFreq : Outport  VectorParamsAs1DForOutWhenUnconnected=off
  stsVal : Outport  Port=2  VectorParamsAs1DForOutWhenUnconnected=off
  wires:
  HDL Counter/1 -> STSFreq/1
  AND/1 -> AND1/1
  HDL Counter1/1 -> Compare To Constant1/1, Compare To Constant/1
  NOT/1 -> HDL Counter1/1
  Compare To Constant/1 -> AND/1
  Compare To Constant1/1 -> AND/2
  preamVal/1 -> NOT/1, AND1/2, HDL Counter1/2
  AND1/1 -> stsVal/1, HDL Counter/1
  STSFreq/1 -> stsFreq/1

== system OFDM_Tx_HW/OFDMTx/IFFT/IFFTValid ==
  preambleValid : Inport
  dataValid : Inport  Port=2
  Switch : Switch  Criteria=u2 ~= 0
  dataIFFTValid : Subsystem
  preambIFFTValid : Subsystem
  ifftValid : Outport  VectorParamsAs1DForOutWhenUnconnected=off
  wires:
  preambleValid/1 -> Switch/2, preambIFFTValid/1(preambValid)
  preambIFFTValid/1(preambIFFTValidOut) -> Switch/1
  dataValid/1 -> dataIFFTValid/1(dataValidIn)
  dataIFFTValid/1(dataIFFTValidOut) -> Switch/3
  Switch/1 -> ifftValid/1

== system OFDM_Tx_HW/OFDMTx/SCMapper/DataMapper ==
  dataIn : Inport
  dataValid : Inport  Port=2
  Delay1 : Delay  DelayLength=80  InitialCondition=0  UseCircularBuffer=on
  Delay2 : Delay  DelayLength=80
  Delay3 : Delay  DelayLength=1  InitialCondition=0  UseCircularBuffer=on
  Delay4 : Delay  DelayLength=80
  Dual Port RAM2 : hdlsllib/HDL RAMs/Dual Port RAM  ram_size=8
      settings: SourceProductBaseCode=SL
  HDL Counter : hdlsllib/Sources/HDL Counter  CountType=Count limited  CountInit=0  CountStep=1  CountMax=159  CountFromType=Initial value  CountFrom=0  CountResetPort=off  CountLoadPort=off  CountEnbPort=on  CountDirPort=off  CountDataType=Unsigned  CountWordLen=8  CountFracLen=0  CountSampTime=1
  HDL Counter1 : hdlsllib/Sources/HDL Counter  CountType=Count limited  CountInit=0  CountStep=1  CountMax=159  CountFromType=Initial value  CountFrom=0  CountResetPort=off  CountLoadPort=off  CountEnbPort=on  CountDirPort=off  CountDataType=Unsigned  CountWordLen=8  CountFracLen=0  CountSampTime=1
  READ_CTRL2 : Subsystem
  Terminator3 : Terminator
  readaddress : Lookup_n-D  NumberOfTableDimensions=1  LookupTableObject=''  BreakpointsForDimension1=[0:159]  BreakpointsForDimension1FirstPoint=10  BreakpointsForDimension2FirstPoint=10  BreakpointsForDimension1Spacing=12  BreakpointsForDimension2Spacing=12  IndexSearchMethod=Evenly spaced points  Table=read_addr_data  TableDataTypeStr=fixdt(0,8,0)  InterpMethod=Flat  DiagnosticForOutOfRangeInput=Error  InternalRulePriority=Speed  OutDataTypeStr=fixdt(0,8,0)  RndMeth=Simplest  InputSameDT=on
  dataOut : Outport  VectorParamsAs1DForOutWhenUnconnected=off
  dataValidOut : Outport  Port=2  VectorParamsAs1DForOutWhenUnconnected=off
  wires:
  READ_CTRL2/1(Out1) -> Dual Port RAM2/4
  Delay3/1 -> Delay2/1
  dataValid/1 -> HDL Counter1/1, Delay1/1, Dual Port RAM2/3
  Dual Port RAM2/2 -> Delay4/1
  Delay1/1 -> READ_CTRL2/2(In2), Delay3/1, HDL Counter/1
  HDL Counter1/1 -> Dual Port RAM2/2
  dataIn/1 -> Dual Port RAM2/1
  HDL Counter/1 -> readaddress/1
  readaddress/1 -> READ_CTRL2/1(In1)
  Dual Port RAM2/1 -> Terminator3/1
  Delay2/1 -> dataValidOut/1
  Delay4/1 -> dataOut/1

== system OFDM_Tx_HW/OFDMTx/SCMapper/PremableMapper ==
  data : Inport
  preambVal : Inport  Port=2
  Delay : Delay  DelayLength=160  InitialCondition=0  UseCircularBuffer=on
  Delay12 : Delay  DelayLength=1  InitialCondition=0  UseCircularBuffer=on
  Dual Port RAM : hdlsllib/HDL RAMs/Dual Port RAM  ram_size=9
      settings: SourceProductBaseCode=SL
  HDL Counter2 : hdlsllib/Sources/HDL Counter  CountType=Count limited  CountInit=0  CountStep=1  CountMax=319  CountFromType=Initial value  CountFrom=0  CountResetPort=off  CountLoadPort=off  CountEnbPort=on  CountDirPort=off  CountDataType=Unsigned  CountWordLen=9  CountFracLen=0  CountSampTime=1
  HDL Counter3 : hdlsllib/Sources/HDL Counter  CountType=Count limited  CountInit=0  CountStep=1  CountMax=319  CountFromType=Initial value  CountFrom=0  CountResetPort=off  CountLoadPort=off  CountEnbPort=on  CountDirPort=off  CountDataType=Unsigned  CountWordLen=9  CountFracLen=0  CountSampTime=1
  READ_CTRL : Subsystem
  Terminator1 : Terminator
  readaddr : Lookup_n-D  NumberOfTableDimensions=1  LookupTableObject=''  BreakpointsForDimension1=0:319  BreakpointsForDimension1FirstPoint=10  BreakpointsForDimension2FirstPoint=10  BreakpointsForDimension1Spacing=12  BreakpointsForDimension2Spacing=12  IndexSearchMethod=Evenly spaced points  Table=read_addr_pream  TableDataTypeStr=fixdt(0,9,0)  InterpMethod=Flat  DiagnosticForOutOfRangeInput=Error  InternalRulePriority=Speed  OutDataTypeStr=fixdt(0,9,0)  RndMeth=Simplest  InputSameDT=on
  preambleShiftOut : Outport  VectorParamsAs1DForOutWhenUnconnected=off
  preambValOut : Outport  Port=2  VectorParamsAs1DForOutWhenUnconnected=off
  wires:
  readaddr/1 -> READ_CTRL/1(In1)
  preambVal/1 -> Delay/1, Dual Port RAM/3, HDL Counter3/1
  READ_CTRL/1(Out1) -> Dual Port RAM/4
  HDL Counter3/1 -> Dual Port RAM/2
  Delay/1 -> READ_CTRL/2(In2), Delay12/1, HDL Counter2/1
  Dual Port RAM/1 -> Terminator1/1
  Delay12/1 -> preambValOut/1
  HDL Counter2/1 -> readaddr/1
  data/1 -> Dual Port RAM/1
  Dual Port RAM/2 -> preambleShiftOut/1

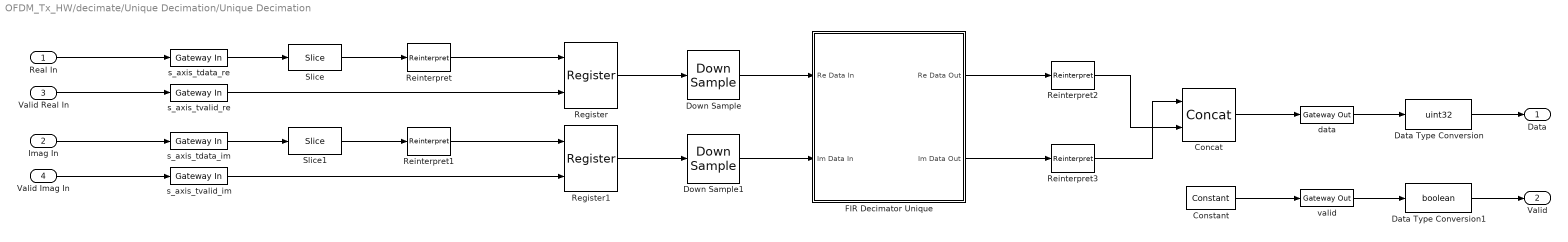
== system OFDM_Tx_HW/decimate/Unique Decimation/Unique Decimation ==
  Real In : Inport
  Imag In : Inport  Port=2
  Valid Real In : Inport  Port=3
  Valid Imag In : Inport  Port=4
  Concat : xbsIndex_r4/Concat  num_inputs=2  dbl_ovrd=off  block_type=concat
  Constant : xbsIndex_r4/Constant  const=1.0  gui_display_data_type=Boolean  arith_type=Boolean  n_bits=16  bin_pt=14  preci_type=Single  exp_width=8  frac_width=24  explicit_period=on  period=1/fs  equ=P=C  opselect=C  inp2=PCIN>>17  opr=+  inp1=P  carry=CIN  dbl_ovrd=off  block_type=constant
  Data Type Conversion : DataTypeConversion  OutDataTypeStr=uint32  ConvertRealWorld=Stored Integer (SI)
  Data Type Conversion1 : DataTypeConversion  OutDataTypeStr=boolean  ConvertRealWorld=Stored Integer (SI)
  Down Sample : xbsIndex_r4/Down Sample  sample_ratio=4  sample_phase="Last Value of Frame  (most efficient)"  en=off  rst=off  latency=1  dbl_ovrd=off  block_type=dsamp
  Down Sample1 : xbsIndex_r4/Down Sample  sample_ratio=4  sample_phase="Last Value of Frame  (most efficient)"  en=off  rst=off  latency=1  dbl_ovrd=off  block_type=dsamp
  FIR Decimator Unique : Subsystem
  Register : xbsIndex_r4/Register  init=0  rst=off  en=on  dbl_ovrd=off  block_type=register
  Register1 : xbsIndex_r4/Register  init=0  rst=off  en=on  dbl_ovrd=off  block_type=register
  Reinterpret : xbsIndex_r4/Reinterpret  force_arith_type=on  arith_type="Signed  (2's comp)"  force_bin_pt=on  bin_pt=14  block_type=reinterpret
  Reinterpret1 : xbsIndex_r4/Reinterpret  force_arith_type=on  arith_type="Signed  (2's comp)"  force_bin_pt=on  bin_pt=14  block_type=reinterpret
  Reinterpret2 : xbsIndex_r4/Reinterpret  force_arith_type=on  arith_type=Unsigned  force_bin_pt=on  bin_pt=0  block_type=reinterpret
  Reinterpret3 : xbsIndex_r4/Reinterpret  force_arith_type=on  arith_type=Unsigned  force_bin_pt=on  bin_pt=0  block_type=reinterpret
  Slice : xbsIndex_r4/Slice  nbits=1  boolean_output=off  mode=Two Bit Locations  bit1=15  base1=LSB of Input  bit0=0  base0=LSB of Input  dbl_ovrd=off  block_type=slice
  Slice1 : xbsIndex_r4/Slice  nbits=1  boolean_output=off  mode=Two Bit Locations  bit1=15  base1=LSB of Input  bit0=0  base0=LSB of Input  dbl_ovrd=off  block_type=slice
  data : xbsIndex_r4/Gateway Out  inherit_from_input=on  hdl_port=on  rows=1  columns=1  UseAsDAC=off  DACChannel='1'  interface=None  automatic_assignment=on  address_offset=hex2dec('00')  intf_name=''  intf_description=''  timing_constraint=None  locs_specified=off  LOCs={}  io_standard={}  block_type=gatewayout
  s_axis_tdata_im : xbsIndex_r4/Gateway In  gui_display_data_type=Fixed-point  arith_type=Unsigned  n_bits=128  bin_pt=0  preci_type=Single  exp_width=8  frac_width=24  rows=1  columns=1  quantization="Round  (unbiased: +/- Inf)"  overflow=Saturate  period=1/fclk  UseAsADC=off  ADCChannel='1'  interface=None  automatic_assignment=on  address_offset=hex2dec('00')  intf_name=''  intf_description=''  default_value=0  timing_constraint=None  locs_specified=off  LOCs={}  io_standard={}  inherit_from_input=off  hdl_port=on  dbl_ovrd=off  block_type=gatewayin
  s_axis_tdata_re : xbsIndex_r4/Gateway In  gui_display_data_type=Fixed-point  arith_type=Unsigned  n_bits=128  bin_pt=0  preci_type=Single  exp_width=8  frac_width=24  rows=1  columns=1  quantization="Round  (unbiased: +/- Inf)"  overflow=Saturate  period=1/fclk  UseAsADC=off  ADCChannel='1'  interface=None  automatic_assignment=on  address_offset=hex2dec('00')  intf_name=''  intf_description=''  default_value=0  timing_constraint=None  locs_specified=off  LOCs={}  io_standard={}  inherit_from_input=off  hdl_port=on  dbl_ovrd=off  block_type=gatewayin
  s_axis_tvalid_im : xbsIndex_r4/Gateway In  gui_display_data_type=Boolean  arith_type=Boolean  n_bits=16  bin_pt=14  preci_type=Single  exp_width=8  frac_width=24  rows=1  columns=1  quantization="Round  (unbiased: +/- Inf)"  overflow=Saturate  period=1/fclk  UseAsADC=off  ADCChannel='1'  interface=None  automatic_assignment=on  address_offset=hex2dec('00')  intf_name=''  intf_description=''  default_value=0  timing_constraint=None  locs_specified=off  LOCs={}  io_standard={}  inherit_from_input=off  hdl_port=on  dbl_ovrd=off  block_type=gatewayin
  s_axis_tvalid_re : xbsIndex_r4/Gateway In  gui_display_data_type=Boolean  arith_type=Boolean  n_bits=16  bin_pt=14  preci_type=Single  exp_width=8  frac_width=24  rows=1  columns=1  quantization="Round  (unbiased: +/- Inf)"  overflow=Saturate  period=1/fclk  UseAsADC=off  ADCChannel='1'  interface=None  automatic_assignment=on  address_offset=hex2dec('00')  intf_name=''  intf_description=''  default_value=0  timing_constraint=None  locs_specified=off  LOCs={}  io_standard={}  inherit_from_input=off  hdl_port=on  dbl_ovrd=off  block_type=gatewayin
  valid : xbsIndex_r4/Gateway Out  inherit_from_input=on  hdl_port=on  rows=1  columns=1  UseAsDAC=off  DACChannel='1'  interface=None  automatic_assignment=on  address_offset=hex2dec('00')  intf_name=''  intf_description=''  timing_constraint=None  locs_specified=off  LOCs={}  io_standard={}  block_type=gatewayout
  Data : Outport
  Valid : Outport  Port=2
  wires:
  Data Type Conversion1/1 -> Valid/1
  Data Type Conversion/1 -> Data/1
  Concat/1 -> data/1
  Reinterpret2/1 -> Concat/2
  Reinterpret3/1 -> Concat/1
  FIR Decimator Unique/2(Im Data Out) -> Reinterpret3/1
  FIR Decimator Unique/1(Re Data Out) -> Reinterpret2/1
  Constant/1 -> valid/1
  Real In/1 -> s_axis_tdata_re/1
  data/1 -> Data Type Conversion/1
  Reinterpret1/1 -> Register1/1
  s_axis_tdata_re/1 -> Slice/1
  Down Sample1/1 -> FIR Decimator Unique/2(Im Data In)
  Valid Real In/1 -> s_axis_tvalid_re/1
  Down Sample/1 -> FIR Decimator Unique/1(Re Data In)
  Imag In/1 -> s_axis_tdata_im/1
  Slice1/1 -> Reinterpret1/1
  Register1/1 -> Down Sample1/1
  s_axis_tvalid_im/1 -> Register1/2
  Reinterpret/1 -> Register/1
  valid/1 -> Data Type Conversion1/1
  Slice/1 -> Reinterpret/1
  s_axis_tvalid_re/1 -> Register/2
  s_axis_tdata_im/1 -> Slice1/1
  Valid Imag In/1 -> s_axis_tvalid_im/1
  Register/1 -> Down Sample/1

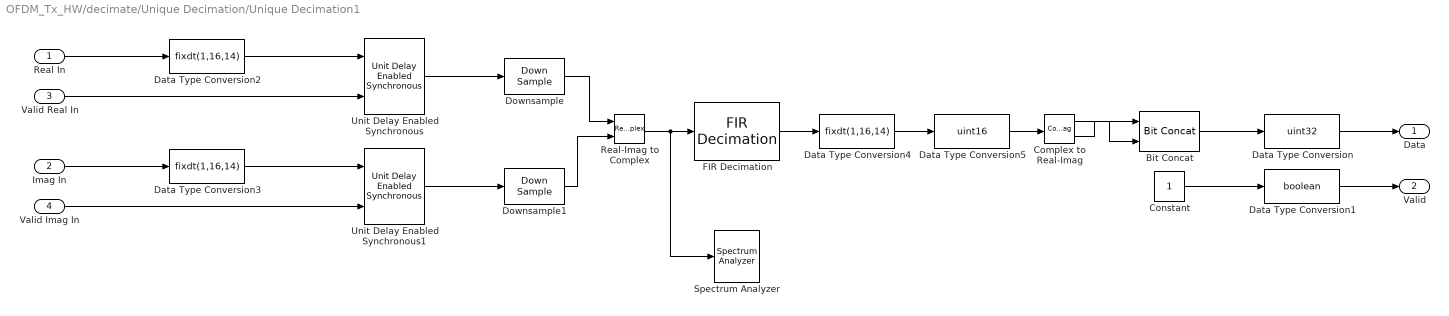
== system OFDM_Tx_HW/decimate/Unique Decimation/Unique Decimation1 ==
  Real In : Inport
  Imag In : Inport  Port=2
  Valid Real In : Inport  Port=3
  Valid Imag In : Inport  Port=4
  Bit Concat : hdlsllib/Logic and Bit Operations/Bit Concat  numInputs=2
  Complex to Real-Imag : ComplexToRealImag
  Constant : Constant  OutDataTypeStr=boolean  SampleTime=1/1e6
  Data Type Conversion : DataTypeConversion  OutDataTypeStr=uint32  ConvertRealWorld=Stored Integer (SI)
  Data Type Conversion1 : DataTypeConversion  OutDataTypeStr=boolean  ConvertRealWorld=Stored Integer (SI)
  Data Type Conversion2 : DataTypeConversion  OutDataTypeStr=fixdt(1,16,14)  ConvertRealWorld=Stored Integer (SI)
  Data Type Conversion3 : DataTypeConversion  OutDataTypeStr=fixdt(1,16,14)  ConvertRealWorld=Stored Integer (SI)
  Data Type Conversion4 : DataTypeConversion  OutDataTypeStr=fixdt(1,16,14)  RndMeth=Round  SaturateOnIntegerOverflow=on
  Data Type Conversion5 : DataTypeConversion  OutDataTypeStr=uint16  ConvertRealWorld=Stored Integer (SI)
  Downsample : DownSample  N=4  RateOptions=Allow multirate processing
  Downsample1 : DownSample  N=4  RateOptions=Allow multirate processing
  FIR Decimation : dspmlti4/FIR Decimation  FilterSource=Dialog parameters  h=decimation_unique.getFilters.Stage1.Numerator  D=decimation_unique.getFilters.Stage1.DecimationFactor  filtStruct=Direct form  FilterObject=FDECIM  framing=Allow multirate processing  inputOffset=0  outputBufInitCond=0  roundingMode=Floor  overflowMode=off  firstCoeffDataTypeStr=Inherit: Same word length as input  firstCoeffMin=[]  firstCoeffMax=[]  firstCoeffLastDataTypeStr=Inherit: Same word length as input  outputDataTypeStr=Inherit: Same as accumulator  outputMin=[]  outputMax=[]  outputLastDataTypeStr=Inherit: Same as accumulator
  Real-Imag to Complex : RealImagToComplex
  Spectrum Analyzer : SpectrumAnalyzer
  Unit Delay Enabled Synchronous : hdlsllib/Discrete/Unit Delay Enabled Synchronous  InitialCondition=0.0  SampleTime=-1
      settings: SourceProductBaseCode=SL
  Unit Delay Enabled Synchronous1 : hdlsllib/Discrete/Unit Delay Enabled Synchronous  InitialCondition=0.0  SampleTime=-1
      settings: SourceProductBaseCode=SL
  Data : Outport
  Valid : Outport  Port=2
  wires:
  Constant/1 -> Data Type Conversion1/1
  Bit Concat/1 -> Data Type Conversion/1
  Complex to Real-Imag/2 -> Bit Concat/1
  Complex to Real-Imag/1 -> Bit Concat/2
  Data Type Conversion5/1 -> Complex to Real-Imag/1
  Data Type Conversion4/1 -> Data Type Conversion5/1
  FIR Decimation/1 -> Data Type Conversion4/1
  Real-Imag to Complex/1 -> FIR Decimation/1, Spectrum Analyzer/1
  Downsample1/1 -> Real-Imag to Complex/2
  Downsample/1 -> Real-Imag to Complex/1
  Unit Delay Enabled Synchronous1/1 -> Downsample1/1
  Unit Delay Enabled Synchronous/1 -> Downsample/1
  Imag In/1 -> Data Type Conversion3/1
  Valid Imag In/1 -> Unit Delay Enabled Synchronous1/2
  Data Type Conversion3/1 -> Unit Delay Enabled Synchronous1/1
  Data Type Conversion2/1 -> Unit Delay Enabled Synchronous/1
  Valid Real In/1 -> Unit Delay Enabled Synchronous/2
  Real In/1 -> Data Type Conversion2/1
  Data Type Conversion/1 -> Data/1
  Data Type Conversion1/1 -> Valid/1
